simulink model "saq212s"  (R2017b)
settings: Solver=ode4  StartTime=0.0  StopTime=10.0  FixedStep=0.1  RelTol=1e-3
settings Model: Creator=GPL  LastModifiedBy=GPL

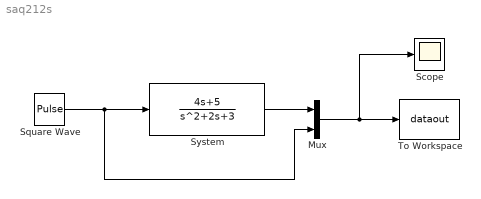
== system saq212s ==
  Mux : Mux  Inputs=2
  Scope : Scope
  Square Wave : DiscretePulseGenerator  PulseType=Time based  Period=5  PulseWidth=50
  System : TransferFcn  Numerator=[4 5]  Denominator=[1 2 3]  ContinuousStateAttributes='Plant'
  To Workspace : ToWorkspace  VariableName=dataout  SaveFormat=Timeseries  SampleTime=-1
  wires:
  Square Wave/1 -> Mux/2, System/1
  System/1 -> Mux/1
  Mux/1 -> Scope/1, To Workspace/1
